simulink model "Parallel"  (R2020b)
settings: Solver=ode4  StartTime=0  StopTime=endtime  MaxStep=0.05  RelTol=1e-5
values from neighbouring files (symbols this model uses):
  Av = 1.545*1.805    (= 2.788725)    [InitiateParallel.m]
  Cd = 0.3    [InitiateParallel.m]
  Cr = 0.0032    [InitiateParallel.m]
  DCT = 1    [InitiateParallel.m]
  Density = (85*19.6e6 + 15*32e6)/100    (= 21460000)    [InitiateParallel.m]
  Eta_gen = 0.6    [InitiateParallel.m]
  EtaEM = Eta    [CreateEMmap.m]
  EtaGEAR = 0.97    [InitiateParallel.m]
  EtaICE = EtaICE_HeavyDIESEL    [InitiateParallel.m]
  EtaPE = 0.98    [InitiateParallel.m]
  grav = 9.81    [InitiateParallel.m]
  ksoc = max(Wbatt)/400/Tau_charge    [InitiateParallel.m]
  ksoc_vect = ksoc*tan(pi/2.05*[-1:1/15:1])*2    [InitiateParallel.m]
  Mv = 40000    [InitiateParallel.m]
  Number_of_gears = 12    [InitiateParallel.m]
  Paux = 3000    [InitiateParallel.m]
  Pem_max = 300000    [InitiateParallel.m]    (also in ParallelBatch_2D.m = EMpower_vector(loop2))
  Pice_max = 300000    [InitiateParallel.m]
  PtoT = zeros(length(P),4)    [CreateICEmap.m]
  rho_air = 1.2    [InitiateParallel.m]
  rw = 0.506    [InitiateParallel.m]
  SOC_batt_ref_value = 70    [InitiateParallel.m]
  SOC_batt_start_value = 100    [InitiateParallel.m]    (also in ParallelBatch_1D.m = SOC(length(SOC(:,1)),2))
  SOC_tract_max = 98    [InitiateParallel.m]
  SOC_tract_min = 12    [InitiateParallel.m]
  Tau_charge = 2    [InitiateParallel.m]
  Tem = Tem_max.*Tref/max(Tref)    [CreateEMmap.m]
  Tem_lim = min([Tem_max*ones(1,length(Wem)); Pem_max./Wem])    [CreateEMmap.m]
  Tem_max = Pem_max/(wice_max/fwr)    (= 2406.42273955)    [InitiateParallel.m]
  Tice_max = Pice_max/(wice_max*row/(length(EtaICE)-1))    [InitiateParallel.m]
  utvx_max = wice_max/((vmax/5)/rw)    (= 26.4940980453)    [InitiateParallel.m]
  Utvx_vect = zeros(1,Number_of_gears+1)    [InitiateParallel.m]
  Wbatt = 8.9*3.6e6    (= 32040000)    [InitiateParallel.m]
  Wem = wem_max.*w/max(w)    [CreateEMmap.m]
  wem_max = wice_max    (= 261.799387799)    [InitiateParallel.m]
  wice_max = 2500*2*pi/60    (= 261.799387799)    [InitiateParallel.m]
  wice_min = 700*2*pi/60    (= 73.3038285838)    [InitiateParallel.m]
undefined symbols (not defined in the file or in its folder): EtaBATT, FuelConsICE, Pbatt, Pbatt_max_new, Pice_max_parallel, Tice, Tlim_ice, Wice
libraries: simulink_need_slupdate x1, simulink x1
(part 2 of 2)

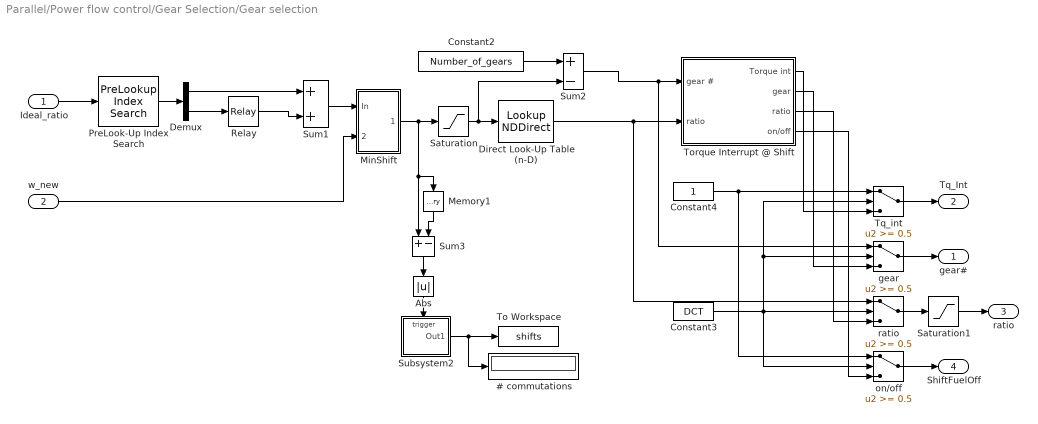
== system Parallel/Power flow control/Gear Selection/Gear selection ==
  Ideal_ratio : Inport
  w_new : Inport  Port=2
  # commutations : Display
  Abs : Abs  SaturateOnIntegerOverflow=on
  Constant2 : Constant  Value=Number_of_gears
  Constant3 : Constant  Value=DCT
  Constant4 : Constant
  Demux : Demux  Outputs=2
      settings: DisplayOption=none
  Direct Look-Up Table (n-D) : LookupNDDirect  NumberOfTableDimensions=1  Table=Utvx_vect
  Memory1 : Memory
  MinShift : Subsystem
  PreLook-Up Index Search : simulink_need_slupdate/PreLookup Index Search  bpData=Utvx_vect  searchMode=Binary Search  cacheBpFlag=off  outputFlag=off  IndexDataType=uint32  extrapMode=Linear Extrapolation  rangeErrorMode=None
      settings: SourceProductBaseCode=SL
  Relay : Relay  OnSwitchValue=0.52  OffSwitchValue=0.48
  Saturation : Saturate  UpperLimit=Number_of_gears-1  LowerLimit=0
  Saturation1 : Saturate  UpperLimit=max(Utvx_vect)  LowerLimit=min(Utvx_vect)
  Subsystem2 : Subsystem  TreatAsAtomicUnit=on
  Sum1 : Sum  SaturateOnIntegerOverflow=on
  Sum2 : Sum  Inputs=+-  SaturateOnIntegerOverflow=on
  Sum3 : Sum  Inputs=+-  SaturateOnIntegerOverflow=on
  To Workspace : ToWorkspace  VariableName=shifts  SampleTime=-1
  Torque Interrupt @ Shift : Subsystem
  Tq_int : Switch  Threshold=0.5  SaturateOnIntegerOverflow=on
  "gear " : Switch  Threshold=0.5  SaturateOnIntegerOverflow=on
  "on/off " : Switch  Threshold=0.5  SaturateOnIntegerOverflow=on
  "ratio " : Switch  Threshold=0.5  SaturateOnIntegerOverflow=on
  gear# : Outport  VectorParamsAs1DForOutWhenUnconnected=off
  Tq_Int : Outport  Port=2  VectorParamsAs1DForOutWhenUnconnected=off
  ratio : Outport  Port=3  VectorParamsAs1DForOutWhenUnconnected=off
  ShiftFuelOff : Outport  Port=4  VectorParamsAs1DForOutWhenUnconnected=off
  wires:
  Ideal_ratio/1 -> PreLook-Up Index Search/1
  w_new/1 -> MinShift/2(Wice_new)
  PreLook-Up Index Search/1 -> Demux/1
  Demux/2 -> Relay/1
  Relay/1 -> Sum1/2
  Direct Look-Up Table (n-D)/1 -> Torque Interrupt @ Shift/2(ratio), "ratio "/1
  Constant2/1 -> Sum2/1
  Sum2/1 -> Torque Interrupt @ Shift/1(gear #), "gear "/1
  Saturation/1 -> Direct Look-Up Table (n-D)/1, Sum2/2
  Torque Interrupt @ Shift/1(Torque int) -> Tq_int/3
  Torque Interrupt @ Shift/2(gear) -> "gear "/3
  Torque Interrupt @ Shift/4(on/off) -> "on/off "/3
  Torque Interrupt @ Shift/3("ratio ") -> "ratio "/3
  Constant3/1 -> Tq_int/2, "gear "/2, "ratio "/2, "on/off "/2
  Constant4/1 -> Tq_int/1, "on/off "/1
  Tq_int/1 -> Tq_Int/1
  "gear "/1 -> gear#/1
  "ratio "/1 -> Saturation1/1
  "on/off "/1 -> ShiftFuelOff/1
  Subsystem2/1(Out1) -> # commutations/1, To Workspace/1
  Memory1/1 -> Sum3/2
  Sum3/1 -> Abs/1
  Abs/1 -> Subsystem2/Trigger
  MinShift/1(Out) -> Sum3/1, Memory1/1, Saturation/1
  Sum1/1 -> MinShift/1(In)
  Saturation1/1 -> ratio/1
  Demux/1 -> Sum1/1

== system Parallel/Power flow control/Optimal operating point/LP-filter ==
  P ice* : Inport
  Gain2 : Gain  Gain=1/(Tau_charge)  SaturateOnIntegerOverflow=on  OutDataTypeStr=Inherit: Same as input  ParamDataTypeStr=Inherit: Same as input
  Sum3 : Sum  Inputs=+-  InputSameDT=on  SaturateOnIntegerOverflow=on  OutDataTypeStr=Inherit: Same as first input
  Wbatt : Integrator  UpperSaturationLimit=Pice_max_parallel  LowerSaturationLimit=0
  P ice : Outport  InitialOutput=0  VectorParamsAs1DForOutWhenUnconnected=off
  wires:
  P ice*/1 -> Sum3/1
  Sum3/1 -> Gain2/1
  Gain2/1 -> Wbatt/1
  Wbatt/1 -> Sum3/2, P ice/1

== system Parallel/Power flow control/Gear Selection/Gear selection/MinShift ==
  In : Inport
  Wice_new : Inport  Port=2
  Abs1 : Abs  SaturateOnIntegerOverflow=on
  Memory2 : Memory
  Memory4 : Memory
  Pulse Generator : DiscretePulseGenerator  Period=4  PulseWidth=2  SampleTime=0.1
  Scope1 : Scope
  Sum4 : Sum  Inputs=+++  SaturateOnIntegerOverflow=on
  Sum5 : Sum  Inputs=+-  SaturateOnIntegerOverflow=on
  ref time : Subsystem  AncestorBlock=|  TreatAsAtomicUnit=on
      | simulink/Model-Wide
      | Utilities/Trigger-Based
      | Linearization
  w<xx : Relay  OnSwitchValue=wice_min*1.2  OffSwitchValue=wice_min*1.1  OnOutputValue=0  OffOutputValue=1
  w>yy : Relay  OnSwitchValue=wice_max*0.66  OffSwitchValue=wice_max*0.65
  Out : Outport  VectorParamsAs1DForOutWhenUnconnected=off
  wires:
  w>yy/1 -> Sum4/2
  w<xx/1 -> Sum4/3
  Pulse Generator/1 -> Scope1/1, Sum4/1
  Memory2/1 -> Sum5/2
  Sum5/1 -> Abs1/1
  Wice_new/1 -> w>yy/1, w<xx/1
  In/1 -> ref time/1(in)
  ref time/1(out) -> Out/1
  Memory4/1 -> Sum5/1, Memory2/1
  Sum4/1 -> Memory4/1
  Abs1/1 -> ref time/Trigger

== system Parallel/Power flow control/Gear Selection/Gear selection/Subsystem2 ==
  Trigger : TriggerPort  TriggerType=either  VariantControl=Variant
  Constant : Constant
  Memory : Memory  InheritSampleTime=on
  Sum : Sum  InputSameDT=on  SaturateOnIntegerOverflow=on  OutDataTypeStr=Inherit: Same as first input
  Out1 : Outport  VectorParamsAs1DForOutWhenUnconnected=off
  wires:
  Sum/1 -> Memory/1, Out1/1
  Memory/1 -> Sum/2
  Constant/1 -> Sum/1

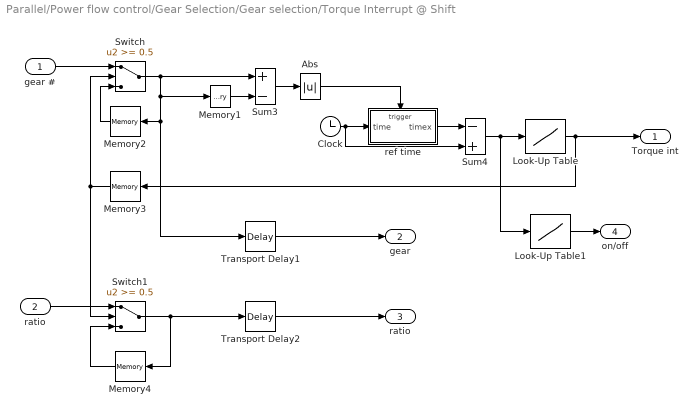
== system Parallel/Power flow control/Gear Selection/Gear selection/Torque Interrupt @ Shift ==
  gear # : Inport
  ratio : Inport  Port=2
  Abs : Abs  SaturateOnIntegerOverflow=on
  Clock : Clock
  Look-Up Table : Lookup  InputValues=[0 0.2 0.8 1.0]  Table=[1 0 0 1]  LookUpMeth=Interpolation-Use End Values  SaturateOnIntegerOverflow=on
  Look-Up Table1 : Lookup  InputValues=[0 0.2 0.2+eps 0.8-eps 0.8 1.0]  Table=[1 1 0 0 1 1]  LookUpMeth=Interpolation-Use End Values  SaturateOnIntegerOverflow=on
  Memory1 : Memory
  Memory2 : Memory  InheritSampleTime=on
  Memory3 : Memory  InheritSampleTime=on
  Memory4 : Memory  InheritSampleTime=on
  Sum3 : Sum  Inputs=+-  SaturateOnIntegerOverflow=on
  Sum4 : Sum  Inputs=-+  SaturateOnIntegerOverflow=on
  Switch : Switch  Threshold=0.5  SaturateOnIntegerOverflow=on
  Switch1 : Switch  Threshold=0.5  SaturateOnIntegerOverflow=on
  Transport Delay1 : TransportDelay  DelayTime=0.6
  Transport Delay2 : TransportDelay  DelayTime=0.6
  ref time : Subsystem  AncestorBlock=|  TreatAsAtomicUnit=on
      | simulink/Model-Wide
      | Utilities/Trigger-Based
      | Linearization
  Torque int : Outport  VectorParamsAs1DForOutWhenUnconnected=off
  gear : Outport  Port=2  VectorParamsAs1DForOutWhenUnconnected=off
  "ratio " : Outport  Port=3  VectorParamsAs1DForOutWhenUnconnected=off
  on/off : Outport  Port=4  VectorParamsAs1DForOutWhenUnconnected=off
  wires:
  Memory1/1 -> Sum3/2
  Sum3/1 -> Abs/1
  Abs/1 -> ref time/Trigger
  Clock/1 -> ref time/1(time), Sum4/2
  Sum4/1 -> Look-Up Table/1, Look-Up Table1/1
  ref time/1(timex) -> Sum4/1
  Look-Up Table/1 -> Torque int/1, Memory3/1
  gear #/1 -> Switch/1
  Switch/1 -> Sum3/1, Memory2/1, Transport Delay1/1, Memory1/1
  Transport Delay1/1 -> gear/1
  Memory2/1 -> Switch/3
  Memory3/1 -> Switch/2, Switch1/2
  ratio/1 -> Switch1/1
  Switch1/1 -> Memory4/1, Transport Delay2/1
  Memory4/1 -> Switch1/3
  Transport Delay2/1 -> "ratio "/1
  Look-Up Table1/1 -> on/off/1

== system Parallel/Power flow control/Gear Selection/Gear selection/MinShift/ref time ==
  in : Inport
  Trigger : TriggerPort  TriggerType=either  VariantControl=Variant
  Zero-Order Hold : ZeroOrderHold  SampleTime=-1
  out : Outport  VectorParamsAs1DForOutWhenUnconnected=off
  wires:
  in/1 -> Zero-Order Hold/1
  Zero-Order Hold/1 -> out/1

== system Parallel/Power flow control/Gear Selection/Gear selection/Torque Interrupt @ Shift/ref time ==
  time : Inport
  Trigger : TriggerPort  VariantControl=Variant
  Zero-Order Hold : ZeroOrderHold  SampleTime=-1
  timex : Outport  VectorParamsAs1DForOutWhenUnconnected=off
  wires:
  time/1 -> Zero-Order Hold/1
  Zero-Order Hold/1 -> timex/1
